simulink model "W02_I_pseudo_derivative"  (R2024b)
settings: Solver=ode4  StartTime=0  StopTime=pd_T  FixedStep=h  RelTol=1e-3
StopFcn:
  | W02_pd_plot;
undefined symbols (not defined in the file or in its folder): pd_Kd, pd_Kp, pd_N1, pd_N2, pd_r, pd_t1, pd_ts
libraries: simulink x1
settings Model: Creator=admin  LastModifiedBy=admin
settings DataIOCC: ReturnWorkspaceOutputs=off

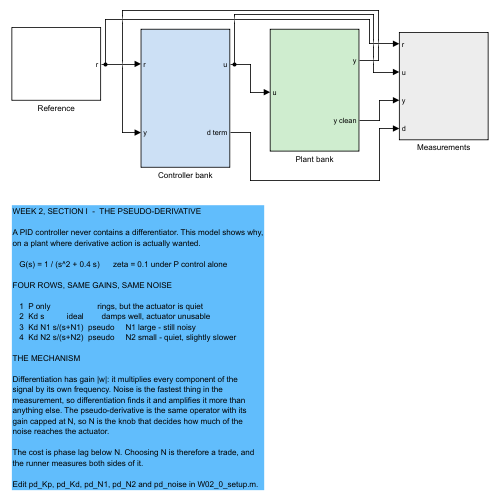
[thumbnail: Simulink's stored preview of the top-level diagram]
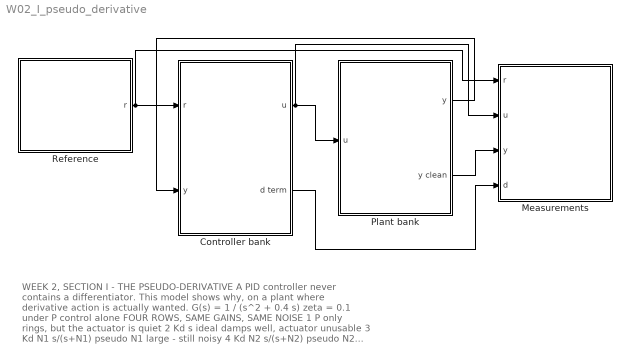
== system W02_I_pseudo_derivative ==
  note: WEEK 2, SECTION I  -  THE PSEUDO-DERIVATIVE
      |
      | A PID controller never contains a differentiator. This model shows why,
      | on a plant where derivative action is actually wanted.
      |
      |    G(s) = 1 / (s^2 + 0.4 s)      zeta = 0.1 under P control alone
      |
      | FOUR ROWS, SAME GAINS, SAME NOISE
      |
      |    1  P only                     rings, but the actuator is quiet
      |    2  Kd s          ideal        damps well, actuator unusable
      |    3  Kd N1 s/(s+N1)  pseudo     N1 large - still noisy
      |    4  Kd N2 s/(s+N2)  pseudo     N2 small - quiet, slightly slower
      |
      | THE MECHANISM
      |
      | Differentiation has gain |w|: it multiplies every component of the
      | signal by its own frequency. Noise is the fastest thing in the
      | measurement, so differentiation finds it and amplifies it more than
      | anything else. The pseudo-derivative is the same operator with its
      | gain capped at N, so N is the knob that decides how much of the
      | noise reaches the actuator.
      |
      | The cost is phase lag below N. Choosing N is therefore a trade, and
      | the runner measures both sides of it.
      |
      | Edit pd_Kp, pd_Kd, pd_N1, pd_N2 and pd_noise in W02_0_setup.m.
  Controller bank : Subsystem
  Measurements : Subsystem
  Plant bank : Subsystem
  Reference : Subsystem
  wires:
  Reference/1(r) -> Controller bank/1(r), Measurements/1(r)
  Controller bank/1(u) -> Plant bank/1(u), Measurements/2(u)
  Plant bank/1(y) -> Controller bank/2(y)
  Plant bank/2(y clean) -> Measurements/3(y)
  Controller bank/2(d term) -> Measurements/4(d)

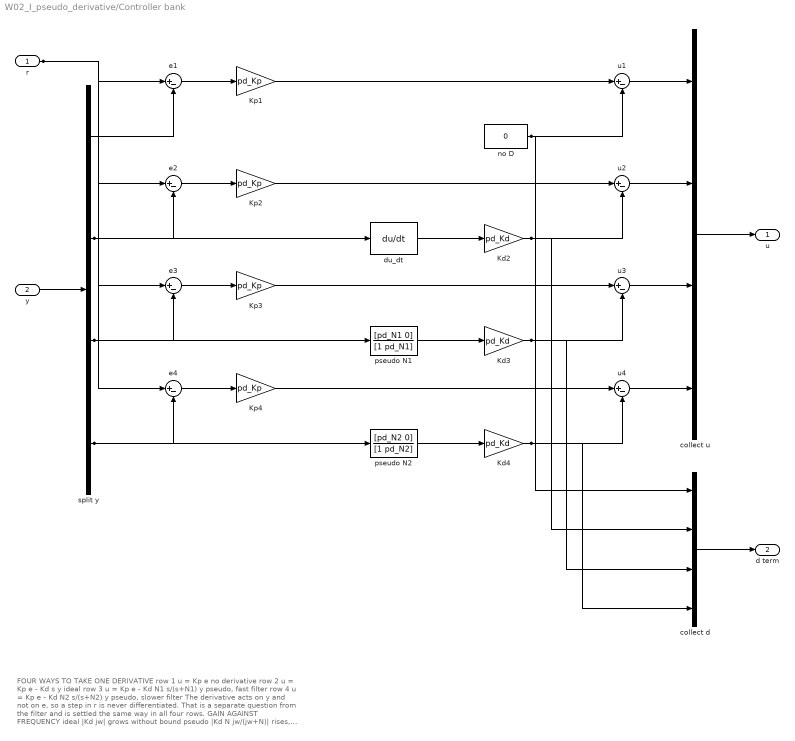
== system W02_I_pseudo_derivative/Controller bank ==
  note: FOUR WAYS TO TAKE ONE DERIVATIVE
      |
      |    row 1   u = Kp e                          no derivative
      |    row 2   u = Kp e - Kd  s        y         ideal
      |    row 3   u = Kp e - Kd  N1 s/(s+N1)  y     pseudo, fast filter
      |    row 4   u = Kp e - Kd  N2 s/(s+N2)  y     pseudo, slower filter
      |
      | The derivative acts on y and not on e, so a step in r is never
      | differentiated. That is a separate question from the filter and is
      | settled the same way in all four rows.
      |
      | GAIN AGAINST FREQUENCY
      |
      |    ideal        |Kd jw|            grows without bound
      |    pseudo       |Kd N jw/(jw+N)|   rises, then levels off at Kd N
      |
      | Below N the two agree. Above N the ideal keeps climbing and the pseudo
      | stops. Measurement noise lives above N, which is the whole point:
      | N chooses how much of the noise reaches the actuator.
  r : Inport
  y : Inport  Port=2
  Kd2 : Gain  Gain=pd_Kd
  Kd3 : Gain  Gain=pd_Kd
  Kd4 : Gain  Gain=pd_Kd
  Kp{1..4} (4 alike) : Gain  Gain=pd_Kp
  collect d : Mux
  collect u : Mux
  du_dt : Derivative
  e{1..4} (4 alike) : Sum  Inputs=|+-
  no D : Constant  Value=0
  pseudo N1 : TransferFcn  Numerator=[pd_N1 0]  Denominator=[1 pd_N1]
  pseudo N2 : TransferFcn  Numerator=[pd_N2 0]  Denominator=[1 pd_N2]
  split y : Demux
  u{1..4} (4 alike) : Sum  Inputs=|+-
  u : Outport
  d term : Outport  Port=2
  wires:
  collect u/1 -> u/1
  collect d/1 -> d term/1
  y/1 -> split y/1
  r/1 -> e1/1, e2/1, e3/1, e4/1
  split y/1 -> e1/2
  e1/1 -> Kp1/1
  Kp1/1 -> u1/1
  u1/1 -> collect u/1
  split y/2 -> e2/2, du_dt/1
  e2/1 -> Kp2/1
  Kp2/1 -> u2/1
  u2/1 -> collect u/2
  split y/3 -> e3/2, pseudo N1/1
  e3/1 -> Kp3/1
  Kp3/1 -> u3/1
  u3/1 -> collect u/3
  split y/4 -> e4/2, pseudo N2/1
  e4/1 -> Kp4/1
  Kp4/1 -> u4/1
  u4/1 -> collect u/4
  no D/1 -> u1/2, collect d/1
  du_dt/1 -> Kd2/1
  Kd2/1 -> u2/2, collect d/2
  pseudo N1/1 -> Kd3/1
  Kd3/1 -> u3/2, collect d/3
  pseudo N2/1 -> Kd4/1
  Kd4/1 -> u4/2, collect d/4

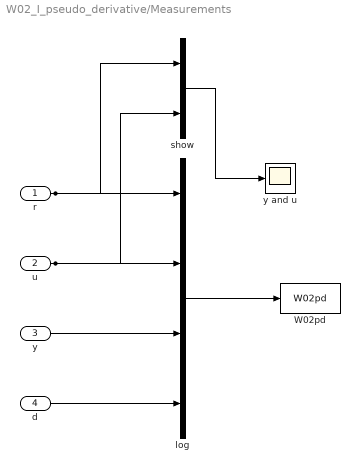
== system W02_I_pseudo_derivative/Measurements ==
  r : Inport
  u : Inport  Port=2
  y : Inport  Port=3
  d : Inport  Port=4
  W02pd : ToWorkspace  VariableName=W02pd  SaveFormat=Structure With Time  SampleTime=-1
  log : Mux
  show : Mux  Inputs=2
  y and u : Scope
  wires:
  r/1 -> log/1, show/1
  u/1 -> log/2, show/2
  y/1 -> log/3
  d/1 -> log/4
  log/1 -> W02pd/1
  show/1 -> y and u/1

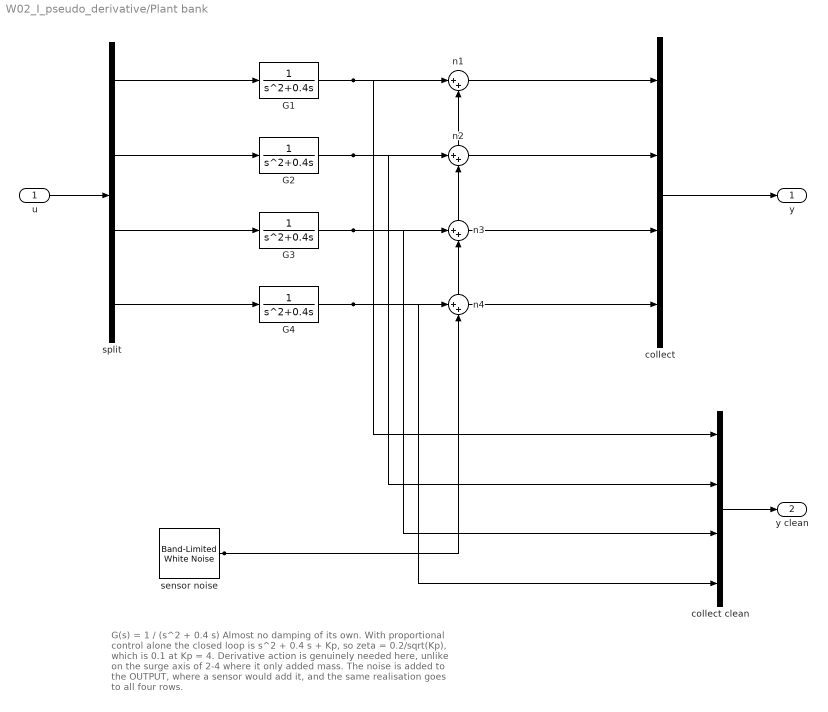
== system W02_I_pseudo_derivative/Plant bank ==
  note: G(s) = 1 / (s^2 + 0.4 s)
      |
      | Almost no damping of its own. With proportional control alone the
      | closed loop is s^2 + 0.4 s + Kp, so zeta = 0.2/sqrt(Kp), which is
      | 0.1 at Kp = 4. Derivative action is genuinely needed here, unlike
      | on the surge axis of 2-4 where it only added mass.
      |
      | The noise is added to the OUTPUT, where a sensor would add it, and
      | the same realisation goes to all four rows.
  u : Inport
  G{1..4} (4 alike) : TransferFcn  Denominator=[1 0.4 0]
  collect : Mux
  collect clean : Mux
  n{1..4} (4 alike) : Sum  Inputs=|++
  sensor noise : simulink/Sources/Band-Limited White Noise  Cov=pd_noise  Ts=pd_ts  seed=[23341]
  split : Demux
  y : Outport
  y clean : Outport  Port=2
  wires:
  collect/1 -> y/1
  collect clean/1 -> y clean/1
  u/1 -> split/1
  split/1 -> G1/1
  G1/1 -> n1/1, collect clean/1
  sensor noise/1 -> n1/2, n2/2, n3/2, n4/2
  n1/1 -> collect/1
  split/2 -> G2/1
  G2/1 -> n2/1, collect clean/2
  n2/1 -> collect/2
  split/3 -> G3/1
  G3/1 -> n3/1, collect clean/3
  n3/1 -> collect/3
  split/4 -> G4/1
  G4/1 -> n4/1, collect clean/4
  n4/1 -> collect/4

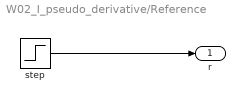
== system W02_I_pseudo_derivative/Reference ==
  step : Step  Time=pd_t1  After=pd_r  SampleTime=0
  r : Outport
  wires:
  step/1 -> r/1
